simulink model "Modelo_PID"  (R2021a)
settings: Solver=VariableStepAuto  StartTime=0.0  StopTime=10.0  MaxStep=0.0001  RelTol=1e-3
values from neighbouring files (symbols this model uses):
  a_cu = 3.9e-3    (= 0.0039)    [Datos.m]
  b_eq = 15.000e-6    (= 1.5e-05)    [Datos.m]
  ba = 0.0113    [Datos.m]
  Cts = 0.818    [Datos.m]
  Id_0 = 0    [Datos.m]
  J_eq = 5.6509e-6    (= 5.6509e-06)    [Datos.m]
  Ksa = 9.0414    [Datos.m]
  Ksia = 2893.2608    [Datos.m]
  lambda_m = 0.01546    [Datos.m]
  Ld = 6.6e-3    (= 0.0066)    [Datos.m]
  Lls = 0.8e-3    (= 0.0008)    [Datos.m]
  Lq = 5.8e-3    (= 0.0058)    [Datos.m]
  Pp = 3.01    [Datos.m]
  r = 314.3008    [Datos.m]
  Rs = 1.02    [Datos.m]
  Rs_ref = 1.02    [Datos.m]
  Rtsamb = 146.7    [Datos.m]
  T_0 = 40.0    (= 40)    [Datos.m]
  T_amb = 40    [Datos.m]
  Ts_ref = 40    [Datos.m]
undefined symbols (not defined in the file or in its folder): R0, Rd, Rq, sigbuilder_block
settings Model: Creator=jpss8  LastModifiedBy=jpss8

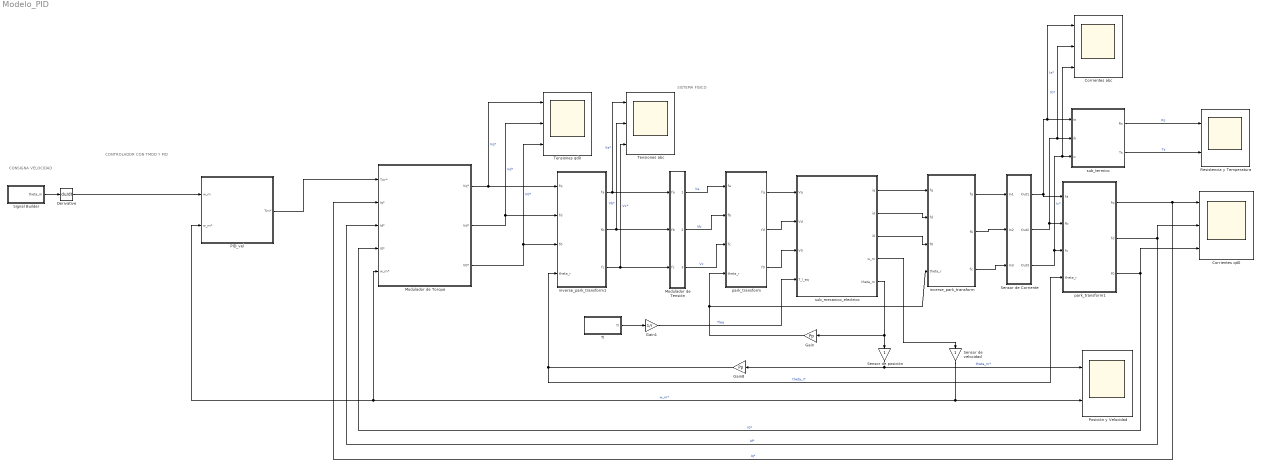
== system Modelo_PID ==
  note: CONTROLADOR CON TMOD Y PID
  note: SISTEMA FÍSICO
  note: CONSIGNA VELOCIDAD
  Corrientes abc : Scope  NumInputPorts=3
  Corrientes qd0 : Scope  NumInputPorts=3
  Derivative : Derivative
  Gain : Gain  Gain=Pp
  Gain1 : Gain  Gain=1/r
  Gain8 : Gain  Gain=Pp
  Modulador de Tensión : Subsystem
  Modulador de Torque : Subsystem
  PID_vel : Subsystem
  Posición y Velocidad : Scope  NumInputPorts=2
  Resistencia y Temperatura : Scope  NumInputPorts=2
  Sensor de Corriente : Subsystem
  Sensor de posición : Gain
  Sensor de velocidad : Gain
  Signal Builder : Subsystem  Tag=STV Subsys  LoadFcn=sigbuilder_block('load',[437.6 199.2 550.4 400 ]);  StartFcn=sigbuilder_block('start');  StopFcn=sigbuilder_block('stop');  ClipboardFcn=sigbuilder_block('clipboard');  mask(Sigbuilder block){tuvar=[0:10]}
      mask help: Simulink:masks:SigbuilderBlock_MD
      mask init:
      | if ~strcmp(get_param(bdroot(gcbh),'SimulationStatus'),'stopped') tuvar = sigbuilder_block('maskInit'); end
      settings: CopyFcn=sigbuilder_block('copy');  DeleteFcn=sigbuilder_block('delete');  ModelCloseFcn=sigbuilder_block('modelClose');  PreSaveFcn=sigbuilder_block('preSave');  PauseFcn=sigbuilder_block('pause');  ContinueFcn=sigbuilder_block('continue');  NameChangeFcn=sigbuilder_block('namechange');  OpenFcn=sigbuilder_block('open',[437.6 199.2 550.4 400 ]);  CloseFcn=sigbuilder_block('close');
      mask Display: plot(0, 0, 100, 100,[2, 2, 32, 32, 2], [68, 8, 8, 68, 68],[32, 2], [38, 38], [32, 19, 2],[53, 60, 44], [32, 17, 17, 2],[16, 16, 31, 31]);txt = getActiveGroup(gcbh);text(2, 100, txt,'verticalAlignment', 'top');
  Tensiones abc : Scope  NumInputPorts=3
  Tensiones qd0 : Scope  NumInputPorts=3
  Tl : Subsystem  Tag=STV Subsys  LoadFcn=sigbuilder_block('load');  StartFcn=sigbuilder_block('start');  StopFcn=sigbuilder_block('stop');  ClipboardFcn=sigbuilder_block('clipboard');  mask(Sigbuilder block){tuvar=[0:10]}
      mask help: Simulink:masks:SigbuilderBlock_MD
      mask init:
      | if ~strcmp(get_param(bdroot(gcbh),'SimulationStatus'),'stopped') tuvar = sigbuilder_block('maskInit'); end
      settings: CopyFcn=sigbuilder_block('copy');  DeleteFcn=sigbuilder_block('delete');  ModelCloseFcn=sigbuilder_block('modelClose');  PreSaveFcn=sigbuilder_block('preSave');  PauseFcn=sigbuilder_block('pause');  ContinueFcn=sigbuilder_block('continue');  NameChangeFcn=sigbuilder_block('namechange');  OpenFcn=sigbuilder_block('open',[5.5 30 1269 678 ]);  CloseFcn=sigbuilder_block('close');
      mask Display: plot(0, 0, 100, 100,[2, 2, 32, 32, 2], [68, 8, 8, 68, 68],[32, 2], [38, 38], [32, 19, 2],[53, 60, 44], [32, 17, 17, 2],[16, 16, 31, 31]);txt = getActiveGroup(gcbh);text(2, 100, txt,'verticalAlignment', 'top');
  inverse_park_transform : MATLAB Function  TreatAsAtomicUnit=on
  inverse_park_transform1 : MATLAB Function  TreatAsAtomicUnit=on
  park_transform : MATLAB Function  TreatAsAtomicUnit=on
  park_transform1 : MATLAB Function  TreatAsAtomicUnit=on
  sub_mecanico_electrico : Subsystem
  sub_termico : Subsystem
  wires:
  Gain1/1 -> sub_mecanico_electrico/4(T_l_eq)  "Tleq"
  Gain/1 -> inverse_park_transform/4(theta_r), park_transform/4(theta_r)
  inverse_park_transform/1(fa) -> Sensor de Corriente/1(In1)
  Derivative/1 -> PID_vel/1(w_m)
  Modulador de Torque/3(V0*) -> inverse_park_transform1/3(f0), Tensiones qd0/3  "V0*"
  inverse_park_transform/2(fb) -> Sensor de Corriente/2(In2)
  sub_mecanico_electrico/4(w_m) -> Sensor de velocidad/1
  PID_vel/1(Tm*) -> Modulador de Torque/1(Tm*')
  sub_termico/2(Ts) -> Resistencia y Temperatura/2  "Ts"
  Sensor de Corriente/2(Out2) -> park_transform1/2(fb), Corrientes abc/2, sub_termico/2(ib)  "Ib*"
  Modulador de Torque/1(Vq*) -> Tensiones qd0/1, inverse_park_transform1/1(fq)  "Vq*"
  inverse_park_transform1/1(fa) -> Tensiones abc/1, Modulador de Tensión/1(fa)  "Va*"
  Modulador de Tensión/3(Out3) -> park_transform/3(fc)  "Vc"
  sub_mecanico_electrico/3(i0) -> inverse_park_transform/3(f0)
  sub_mecanico_electrico/2(id) -> inverse_park_transform/2(fd)
  inverse_park_transform1/2(fb) -> Modulador de Tensión/2(fb), Tensiones abc/2  "Vb*"
  sub_termico/1(Rs) -> Resistencia y Temperatura/1  "Rs"
  park_transform1/2(fd) -> Modulador de Torque/3(Id*), Corrientes qd0/2  "Id*"
  sub_mecanico_electrico/5(theta_m) -> Sensor de posición/1, Gain/1
  Gain8/1 -> park_transform1/4(theta_r), inverse_park_transform1/4(theta_r)  "theta_r*"
  inverse_park_transform1/3(fc) -> Modulador de Tensión/3(fc), Tensiones abc/3  "Vc*"
  Tl/1(Tl) -> Gain1/1
  Sensor de Corriente/1(Out1) -> park_transform1/1(fa), Corrientes abc/1, sub_termico/1(ia)  "Ia*"
  park_transform1/1(fq) -> Modulador de Torque/2(Iq*), Corrientes qd0/1  "Iq*"
  park_transform/3(f0) -> sub_mecanico_electrico/3(V0)
  sub_mecanico_electrico/1(iq) -> inverse_park_transform/1(fq)
  Modulador de Torque/2(Vd*) -> Tensiones qd0/2, inverse_park_transform1/2(fd)  "Vd*"
  Sensor de posición/1 -> Gain8/1, Posición y Velocidad/1  "theta_m*"
  Sensor de Corriente/3(Out3) -> park_transform1/3(fc), Corrientes abc/3, sub_termico/3(ic)  "Ic*"
  park_transform1/3(f0) -> Modulador de Torque/4(I0*), Corrientes qd0/3  "I0*"
  Sensor de velocidad/1 -> PID_vel/2(w_m*), Modulador de Torque/5(w_m*), Posición y Velocidad/2  "w_m*"
  park_transform/2(fd) -> sub_mecanico_electrico/2(Vd)
  park_transform/1(fq) -> sub_mecanico_electrico/1(Vq)
  Modulador de Tensión/2(Out2) -> park_transform/2(fb)  "Vb"
  inverse_park_transform/3(fc) -> Sensor de Corriente/3(In3)
  Modulador de Tensión/1(Out1) -> park_transform/1(fa)  "Va"
  Signal Builder/1(theta_m) -> Derivative/1

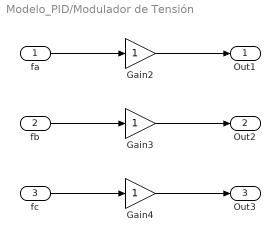
== system Modelo_PID/Modulador de Tensión ==
  fa : Inport
  fb : Inport  Port=2
  fc : Inport  Port=3
  Gain2 : Gain
  Gain3 : Gain
  Gain4 : Gain
  Out1 : Outport
  Out2 : Outport  Port=2
  Out3 : Outport  Port=3
  wires:
  fa/1 -> Gain2/1
  fb/1 -> Gain3/1
  Gain3/1 -> Out2/1
  Gain4/1 -> Out3/1
  fc/1 -> Gain4/1
  Gain2/1 -> Out1/1

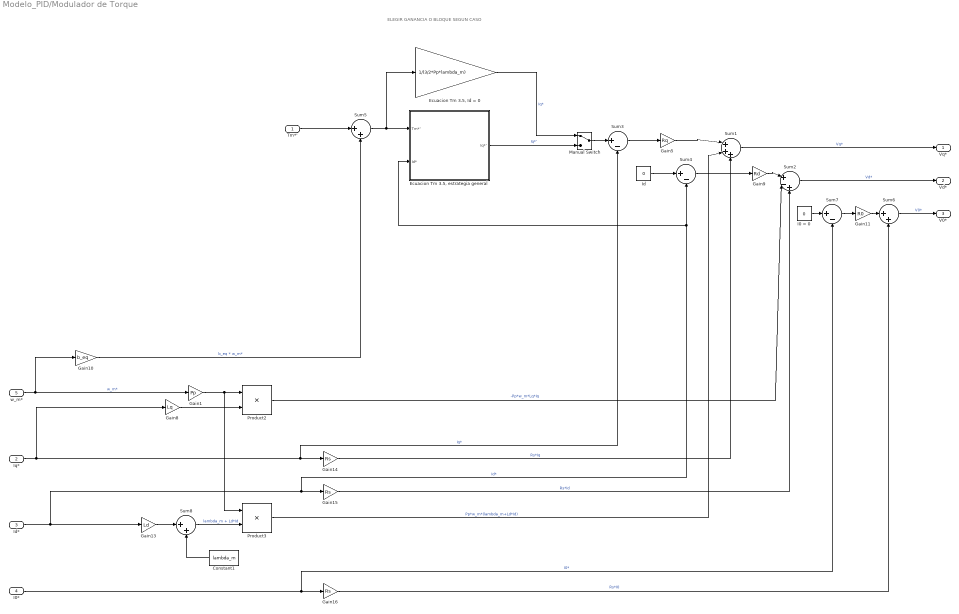
== system Modelo_PID/Modulador de Torque ==
  note: ELEGIR GANANCIA O BLOQUE SEGUN CASO
  Tm*' : Inport
  Iq* : Inport  Port=2
  Id* : Inport  Port=3
  I0* : Inport  Port=4
  w_m* : Inport  Port=5
  Constant1 : Constant  Value=lambda_m
  "Ecuacion Tm 3.5, Id = 0" : Gain  Gain=1/(3/2*Pp*lambda_m)
  "Ecuacion Tm 3.5, estrategia general" : Subsystem
  Gain1 : Gain  Gain=Pp
  Gain10 : Gain  Gain=b_eq
  Gain11 : Gain  Gain=R0
  Gain13 : Gain  Gain=Ld
  Gain14 : Gain  Gain=Rs
  Gain15 : Gain  Gain=Rs
  Gain16 : Gain  Gain=Rs
  Gain5 : Gain  Gain=Rq
  Gain8 : Gain  Gain=Lq
  Gain9 : Gain  Gain=Rd
  I0 = 0 : Constant  Value=0
  Id : Constant  Value=0
  Manual Switch : ManualSwitch
  Product2 : Product
  Product3 : Product
  Sum1 : Sum  Inputs=|+++
  Sum2 : Sum  Inputs=|+-+
  Sum3 : Sum  Inputs=|+-
  Sum4 : Sum  Inputs=|+-
  Sum5 : Sum  Inputs=|++
  Sum6 : Sum  Inputs=|++
  Sum7 : Sum  Inputs=|+-
  Sum8 : Sum  Inputs=|++
  Vq* : Outport
  Vd* : Outport  Port=2
  V0* : Outport  Port=3
  wires:
  Sum7/1 -> Gain11/1
  I0 = 0/1 -> Sum7/1
  "Ecuacion Tm 3.5, estrategia general"/1(Iq*') -> Manual Switch/2  "Iq*'"
  Tm*'/1 -> Sum5/1
  "Ecuacion Tm 3.5, Id = 0"/1 -> Manual Switch/1  "Iq*"
  Sum4/1 -> Gain9/1
  Sum5/1 -> "Ecuacion Tm 3.5, Id = 0"/1, "Ecuacion Tm 3.5, estrategia general"/1(Tm*')
  Id/1 -> Sum4/1
  Gain5/1 -> Sum1/1
  Gain9/1 -> Sum2/1
  Sum3/1 -> Gain5/1
  Sum2/1 -> Vd*/1  "Vd*"
  Gain11/1 -> Sum6/1
  Sum1/1 -> Vq*/1  "Vq*"
  Gain10/1 -> Sum5/2  "b_eq * w_m*"
  Gain14/1 -> Sum1/3  "Rs*Iq"
  Product2/1 -> Sum2/2  "-Pp*w_m*Lq*Iq"
  Gain15/1 -> Sum2/3  "Rs*Id"
  Gain16/1 -> Sum6/2  "Rs*I0"
  Product3/1 -> Sum1/2  "Pp*w_m*(lambda_m+Ld*Id)"
  w_m*/1 -> Gain10/1, Gain1/1  "w_m*"
  Iq*/1 -> Sum3/2, Gain14/1, Gain8/1  "Iq*"
  Gain13/1 -> Sum8/1
  Gain8/1 -> Product2/2
  Gain1/1 -> Product3/1, Product2/1
  Constant1/1 -> Sum8/2
  Sum8/1 -> Product3/2  "lambda_m + Ld*Id"
  Id*/1 -> "Ecuacion Tm 3.5, estrategia general"/2(Id*), Sum4/2, Gain15/1, Gain13/1  "Id*"
  I0*/1 -> Sum7/2, Gain16/1  "I0*"
  Sum6/1 -> V0*/1  "V0*"
  Manual Switch/1 -> Sum3/1

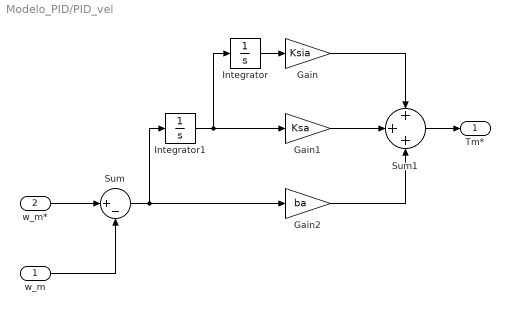
== system Modelo_PID/PID_vel ==
  w_m : Inport
  w_m* : Inport  Port=2
  Gain : Gain  Gain=Ksia
  Gain1 : Gain  Gain=Ksa
  Gain2 : Gain  Gain=ba
  Integrator : Integrator
  Integrator1 : Integrator
  Sum : Sum  Inputs=|+-
  Sum1 : Sum  Inputs=+++
  Tm* : Outport
  wires:
  w_m*/1 -> Sum/1
  Gain1/1 -> Sum1/2
  Sum1/1 -> Tm*/1
  Sum/1 -> Integrator1/1, Gain2/1
  Integrator/1 -> Gain/1
  Gain2/1 -> Sum1/3
  w_m/1 -> Sum/2
  Gain/1 -> Sum1/1
  Integrator1/1 -> Gain1/1, Integrator/1

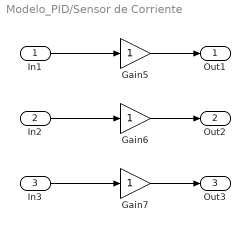
== system Modelo_PID/Sensor de Corriente ==
  In1 : Inport
  In2 : Inport  Port=2
  In3 : Inport  Port=3
  Gain5 : Gain
  Gain6 : Gain
  Gain7 : Gain
  Out1 : Outport
  Out2 : Outport  Port=2
  Out3 : Outport  Port=3
  wires:
  Gain6/1 -> Out2/1
  Gain7/1 -> Out3/1
  In3/1 -> Gain7/1
  Gain5/1 -> Out1/1
  In2/1 -> Gain6/1
  In1/1 -> Gain5/1

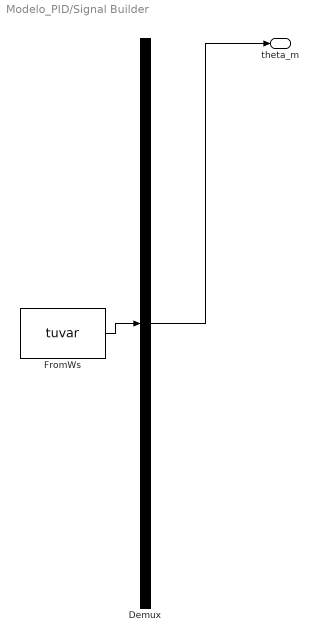
== system Modelo_PID/Signal Builder ==
  Demux : Demux  Tag=STV Demux  Outputs=1
      settings: DisplayOption=none
  FromWs : FromWorkspace  Tag=STV FromWs  VariableName=tuvar
      SigBuilderData=|
      | common.afterFinalStr = 'Extrapolate'
      | common.sampleTime = 0
      | dataSet.timeRange = [0 10]
      | dataSet.name = 'Group 1'
      | sbobj.Groups.Name = 'Group 1'
      | sbobj.Groups.Signals.Name = 'theta_m'
      | sbobj.Groups.Signals.XData = [0 1.24 1.24 9.34 9.34 10]
      | sbobj.Groups.Signals.YData = [0 0 13 200 0 0]
  theta_m : Outport  Tag=STV Outport
  wires:
  Demux/1 -> theta_m/1
  FromWs/1 -> Demux/1

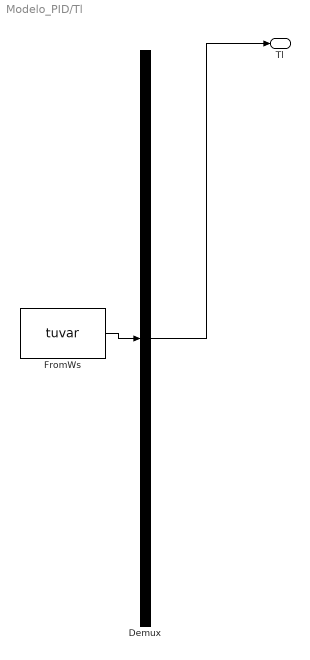
== system Modelo_PID/Tl ==
  Demux : Demux  Tag=STV Demux  Outputs=1
      settings: DisplayOption=none
  FromWs : FromWorkspace  Tag=STV FromWs  VariableName=tuvar
      SigBuilderData=|
      | common.afterFinalStr = 'Extrapolate'
      | common.sampleTime = 0
      | dataSet.timeRange = [0 1]
      | dataSet.name = 'Group 1'
      | sbobj.Groups.Name = 'Group 1'
      | sbobj.Groups.Signals.Name = 'Tl'
      | sbobj.Groups.Signals.XData = [0 0.3 0.3 0.5 0.5 0.9 0.9 1]
      | sbobj.Groups.Signals.YData = [0 0 6.28 6.28 -6.28 -6.28 0 0]
      | sbobj.Groups.TimeRange = [0 1]
  Tl : Outport  Tag=STV Outport
  wires:
  FromWs/1 -> Demux/1
  Demux/1 -> Tl/1

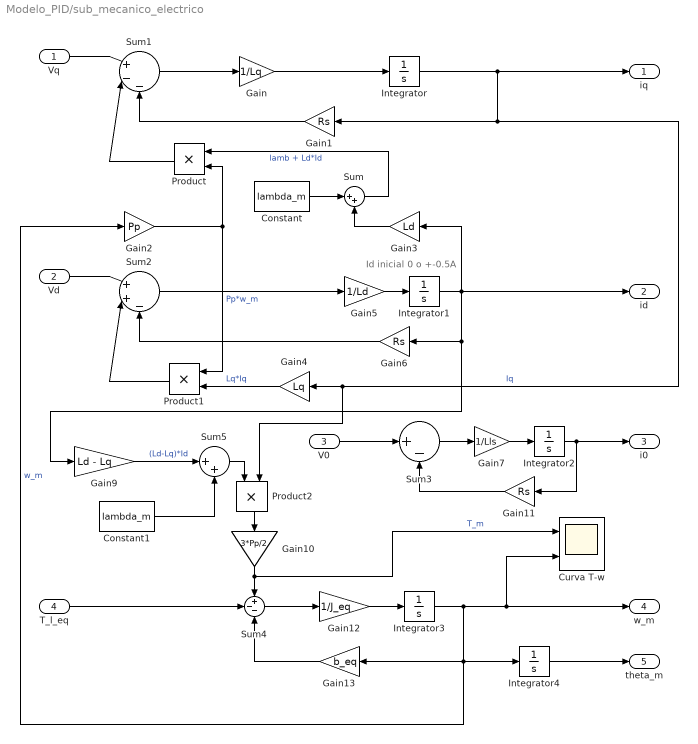
== system Modelo_PID/sub_mecanico_electrico ==
  note: Id inicial 0 o +-0.5A
  Vq : Inport
  Vd : Inport  Port=2
  V0 : Inport  Port=3
  T_l_eq : Inport  Port=4
  Constant : Constant  Value=lambda_m
  Constant1 : Constant  Value=lambda_m
  Curva T-w : Scope  NumInputPorts=2
  Gain : Gain  Gain=1/Lq
  Gain1 : Gain  Gain=Rs
  Gain10 : Gain  Gain=3*Pp/2
  Gain11 : Gain  Gain=Rs
  Gain12 : Gain  Gain=1/J_eq
  Gain13 : Gain  Gain=b_eq
  Gain2 : Gain  Gain=Pp
  Gain3 : Gain  Gain=Ld
  Gain4 : Gain  Gain=Lq
  Gain5 : Gain  Gain=1/Ld
  Gain6 : Gain  Gain=Rs
  Gain7 : Gain  Gain=1/Lls
  Gain9 : Gain  Gain=Ld - Lq
  Integrator{,2..4} (4 alike) : Integrator
  Integrator1 : Integrator  InitialCondition=Id_0
  Product : Product
  Product1 : Product
  Product2 : Product
  Sum : Sum  Inputs=|++
  Sum1 : Sum  Inputs=|+--
  Sum2 : Sum  Inputs=|++-
  Sum3 : Sum  Inputs=|+-
  Sum4 : Sum  Inputs=+--
  Sum5 : Sum  Inputs=|++
  iq : Outport
  id : Outport  Port=2
  i0 : Outport  Port=3
  w_m : Outport  Port=4
  theta_m : Outport  Port=5
  wires:
  Gain12/1 -> Integrator3/1
  T_l_eq/1 -> Sum4/2
  Sum4/1 -> Gain12/1
  Gain10/1 -> Curva T-w/1, Sum4/1  "T_m"
  Integrator4/1 -> theta_m/1
  Gain13/1 -> Sum4/3
  Integrator3/1 -> Gain2/1, Integrator4/1, Gain13/1, Curva T-w/2, w_m/1  "w_m"
  Constant1/1 -> Sum5/2
  Gain9/1 -> Sum5/1  "(Ld-Lq)*Id"
  Sum5/1 -> Product2/1
  Product2/1 -> Gain10/1
  V0/1 -> Sum3/1
  Gain11/1 -> Sum3/2
  Gain5/1 -> Integrator1/1
  Sum2/1 -> Gain5/1
  Integrator1/1 -> Gain9/1, Gain6/1, id/1, Gain3/1
  Product/1 -> Sum1/2
  Integrator2/1 -> i0/1, Gain11/1
  Product1/1 -> Sum2/2
  Gain4/1 -> Product1/2  "Lq*Iq"
  Gain1/1 -> Sum1/3
  Gain6/1 -> Sum2/3
  Sum/1 -> Product/1  "lamb + Ld*Id"
  Sum3/1 -> Gain7/1
  Gain7/1 -> Integrator2/1
  Vd/1 -> Sum2/1
  Gain3/1 -> Sum/2
  Gain2/1 -> Product1/1, Product/2  "Pp*w_m"
  Integrator/1 -> Gain1/1, Gain4/1, Product2/2, iq/1  "Iq"
  Sum1/1 -> Gain/1
  Gain/1 -> Integrator/1
  Constant/1 -> Sum/1
  Vq/1 -> Sum1/1

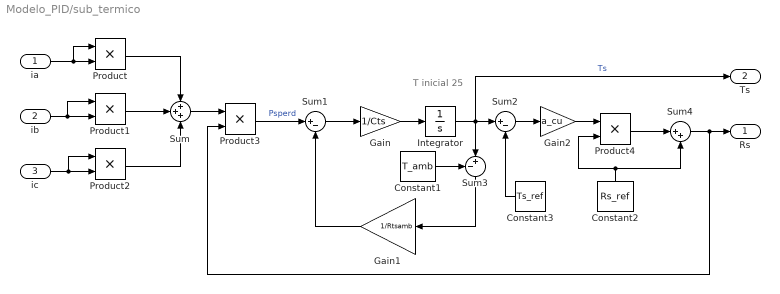
== system Modelo_PID/sub_termico ==
  note: T inicial 25
  ia : Inport
  ib : Inport  Port=2
  ic : Inport  Port=3
  Constant1 : Constant  Value=T_amb
  Constant2 : Constant  Value=Rs_ref
  Constant3 : Constant  Value=Ts_ref
  Gain : Gain  Gain=1/Cts
  Gain1 : Gain  Gain=1/Rtsamb
  Gain2 : Gain  Gain=a_cu
  Integrator : Integrator  InitialCondition=T_0
  Product{,1..4} (5 alike) : Product
  Sum : Sum  Inputs=+++
  Sum1 : Sum  Inputs=|+-
  Sum2 : Sum  Inputs=|+-
  Sum3 : Sum  Inputs=-+|
  Sum4 : Sum  Inputs=|++
  Rs : Outport
  Ts : Outport  Port=2
  wires:
  ic/1 -> Product2/1, Product2/2
  ib/1 -> Product1/1, Product1/2
  ia/1 -> Product/1, Product/2
  Product/1 -> Sum/1
  Product1/1 -> Sum/2
  Product2/1 -> Sum/3
  Product3/1 -> Sum1/1  "Psperd"
  Sum/1 -> Product3/1
  Sum4/1 -> Product3/2, Rs/1
  Gain1/1 -> Sum1/2
  Gain/1 -> Integrator/1
  Sum1/1 -> Gain/1
  Integrator/1 -> Ts/1, Sum3/2, Sum2/1  "Ts"
  Sum3/1 -> Gain1/1
  Constant1/1 -> Sum3/1
  Sum2/1 -> Gain2/1
  Gain2/1 -> Product4/1
  Product4/1 -> Sum4/1
  Constant2/1 -> Product4/2, Sum4/2
  Constant3/1 -> Sum2/2

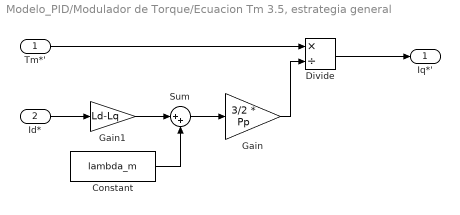
== system Modelo_PID/Modulador de Torque/Ecuacion Tm 3.5, estrategia general ==
  Tm*' : Inport
  Id* : Inport  Port=2
  Constant : Constant  Value=lambda_m
  Divide : Product  Inputs=*/
  Gain : Gain  Gain=3/2 * Pp
  Gain1 : Gain  Gain=Ld-Lq
  Sum : Sum  Inputs=|++
  Iq*' : Outport
  wires:
  Tm*'/1 -> Divide/1
  Id*/1 -> Gain1/1
  Gain1/1 -> Sum/1
  Constant/1 -> Sum/2
  Sum/1 -> Gain/1
  Divide/1 -> Iq*'/1
  Gain/1 -> Divide/2

== matlab function Modelo_PID/inverse_park_transform ==
  data: fq input; fa output; fd input; f0 input; theta_r input; fb output; fc output
function [fa, fb, fc] =  inverse_park_transform(fq, fd, f0, theta_r)

ITP = [cos(theta_r)             sin(theta_r)           1;
       cos(theta_r - 2*pi/3)    sin(theta_r - 2*pi/3)  1;
       cos(theta_r + 2*pi/3)    sin(theta_r + 2*pi/3)  1];

abc = ITP*[fq; fd; f0];

fa = abc(1);
fb = abc(2);
fc = abc(3);
end

== matlab function Modelo_PID/inverse_park_transform1 ==
  data: fq input; fa output; fd input; f0 input; theta_r input; fb output; fc output
function [fa, fb, fc] =  inverse_park_transform(fq, fd, f0, theta_r)

ITP = [cos(theta_r)             sin(theta_r)           1;
       cos(theta_r - 2*pi/3)    sin(theta_r - 2*pi/3)  1;
       cos(theta_r + 2*pi/3)    sin(theta_r + 2*pi/3)  1];

abc = ITP*[fq; fd; f0];

fa = abc(1);
fb = abc(2);
fc = abc(3);
end

== matlab function Modelo_PID/park_transform ==
  data: fa input; fq output; fb input; fc input; theta_r input; fd output; f0 output
function [fq, fd, f0] =  park_transform(fa, fb, fc, theta_r)
    
TP = 2/3*[cos(theta_r)  cos(theta_r - 2*pi/3)   cos(theta_r + 2*pi/3);
          sin(theta_r)  sin(theta_r - 2*pi/3)   sin(theta_r + 2*pi/3);
          1/2           1/2                     1/2];
     
qd0 = TP*[fa; fb; fc];

fq = qd0(1);
fd = qd0(2);
f0 = qd0(3);
end

== matlab function Modelo_PID/park_transform1 ==
  data: fa input; fq output; fb input; fc input; theta_r input; fd output; f0 output
function [fq, fd, f0] =  park_transform(fa, fb, fc, theta_r)
    
TP = 2/3*[cos(theta_r)  cos(theta_r - 2*pi/3)   cos(theta_r + 2*pi/3);
          sin(theta_r)  sin(theta_r - 2*pi/3)   sin(theta_r + 2*pi/3);
          1/2           1/2                     1/2];
     
qd0 = TP*[fa; fb; fc];

fq = qd0(1);
fd = qd0(2);
f0 = qd0(3);
end
